simulink model "Final_SEA_Model"  (R2021a)
settings: Solver=VariableStepAuto  StartTime=0.0  StopTime=10  RelTol=1e-3
values from neighbouring files (symbols this model uses):
  B = 0.015    [Project_reading_1.m]
  C = 0.8    [Project_reading_1.m]
  g = 5    [Project_reading_1.m]
  J = 0.0236    [Project_reading_1.m]
  k = 3    [Project_reading_1.m]
  Ks = 18000    [Project_reading_1.m]
  Kt = 1.78    [Project_reading_1.m]
  L = 0.0063    [Project_reading_1.m]
  m = 8    [Project_reading_1.m]
  P = 1    [Project_reading_1.m]
  R = 2.1975    [Project_reading_1.m]
libraries: simulink_extras x2, pid_lib x1
settings Model: Creator=Panda  LastModifiedBy=Panda
settings ConfigComp: PSVerificationMode=BugFinder  PSAutoStubLUT=on

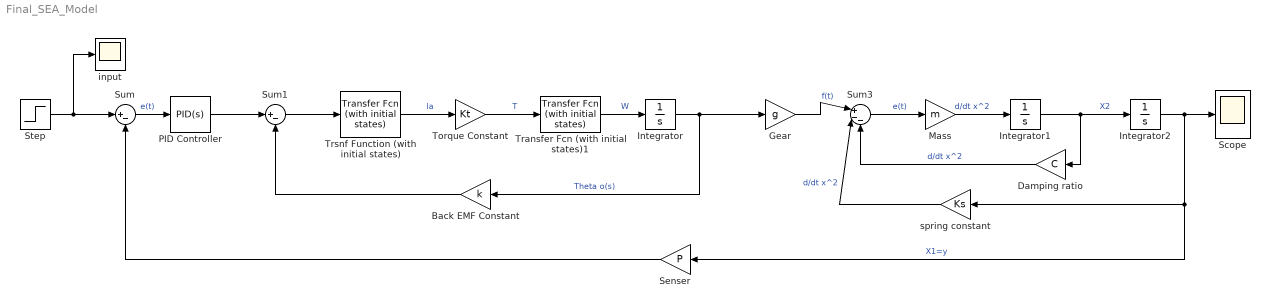
== system Final_SEA_Model ==
  Back EMF Constant : Gain  Gain=k
  Damping ratio : Gain  Gain=C
  Gear : Gain  Gain=g
  Integrator : Integrator
  Integrator1 : Integrator
  Integrator2 : Integrator
  Mass : Gain  Gain=m
  PID Controller : pid_lib/PID Controller  Controller=PID  Form=Parallel  TimeDomain=Continuous-time  UseExternalTs=off  SampleTime=-1  IntegratorMethod=Forward Euler  FilterMethod=Forward Euler  ControllerParametersSource=internal  P=19538.8  I=25686.5  D=2679.99  UseFilter=on  N=100  TunerSelectOption=Transfer Function Based (PID Tuner App)  InitialConditionSource=internal  InitialConditionForIntegrator=0  InitialConditionForFilter=0  DifferentiatorICPrevScaledInput=0  ExternalReset=none  TrackingMode=off  Kt=1  LimitOutput=off  SatLimitsSource=internal  UpperSaturationLimit=inf  LowerSaturationLimit=-inf  LinearizeAsGain=on  AntiWindupMode=none  Kb=1  POutMin=[]  POutMax=[]  IOutMin=[]  IOutMax=[]  DOutMin=[]  DOutMax=[]  NOutMin=[]  NOutMax=[]  SumOutMin=[]  SumOutMax=[]  SaturationOutMin=[]  SaturationOutMax=[]  PParamMin=[]  PParamMax=[]  IParamMin=[]  IParamMax=[]  DParamMin=[]  DParamMax=[]  NParamMin=[]  NParamMax=[]  KbParamMin=[]  KbParamMax=[]  KtParamMin=[]  KtParamMax=[]  KbOutMin=[]  KbOutMax=[]  KtOutMin=[]  KtOutMax=[]  IntegratorOutMin=[]  IntegratorOutMax=[]  FilterOutMin=[]  FilterOutMax=[]  SumI1OutMin=[]  SumI1OutMax=[]  SumI2OutMin=[]  SumI2OutMax=[]  SumI3OutMin=[]  SumI3OutMax=[]  SumI4OutMin=[]  SumI4OutMax=[]  SumDOutMin=[]  SumDOutMax=[]  DifferentiatorOutMin=[]  DifferentiatorOutMax=[]  FilterDiffOutCoefMin=[]  FilterDiffOutCoefMax=[]  ReciprocalOutMin=[]  ReciprocalOutMax=[]  SumDenOutMin=[]  SumDenOutMax=[]  SumNumOutMin=[]  SumNumOutMax=[]  DivideOutMin=[]  DivideOutMax=[]  UdiffTsProdOutMin=[]  UdiffTsProdOutMax=[]  NTsProdOutMin=[]  NTsProdOutMax=[]  UintegralTsProdOutMin=[]  UintegralTsProdOutMax=[]  UngainTsProdOutMin=[]  UngainTsProdOutMax=[]  IntegratorContinuousStateAttributes=''  IntegratorStateMustResolveToSignalObject=off  IntegratorRTWStateStorageClass=Auto  FilterContinuousStateAttributes=''  FilterStateMustResolveToSignalObject=off  FilterRTWStateStorageClass=Auto  ParallelPVariant=InternalParameters  IdealPVariant=Disabled  IVariant=InternalParameters  DVariant=InternalParameters  IntegratorVariant=Continuous  SatVariant=Disabled  AWVariant=Passthrough  PCopyVariant=Disabled  TRVariant=Disabled  FdbkBlocksVariant=Forward  IdealPFdbkVariant=Disabled  SatFdbkVariant=Disabled  DerivativeFilterVariant=ContFilter  NVariant=InternalParameters  NCopyVariant=Disabled  FilterICVariant=InternalICsFilter  IntegratorICVariant=InternalICs  ExternalResetVariant=Disabled  TRSumVariant=Passthrough  SumFdbkVariant=Disabled  SumVariant=Sum_PID  TsampFilterVariant=InternalTs  TsampNgainVariant=Passthrough  TsampIntegralVariant=Passthrough  ExternalSaturationOutDataTypeStr=Inherit: Same as second input
  Scope : Scope
  Senser : Gain  Gain=P
  Step : Step  Time=0  SampleTime=0
  Sum : Sum  Inputs=|+-
  Sum1 : Sum  Inputs=|+-
  Sum3 : Sum  Inputs=|+--
  Torque Constant : Gain  Gain=Kt
  Transfer Fcn (with initial states)1 : simulink_extras/Additional Linear/Transfer Fcn (with initial states)  N=[1]  D="[J  B]"  X0=.5
  Trsnf Function (with initial states) : simulink_extras/Additional Linear/Transfer Fcn (with initial states)  N=[1]  D="[L  R]"  X0=.5
  input : Scope
  spring constant : Gain  Gain=Ks
  wires:
  Trsnf Function (with initial states)/1 -> Torque Constant/1  "la"
  Torque Constant/1 -> Transfer Fcn (with initial states)1/1  "T"
  Sum1/1 -> Trsnf Function (with initial states)/1
  Back EMF Constant/1 -> Sum1/2
  Step/1 -> input/1, Sum/1
  Transfer Fcn (with initial states)1/1 -> Integrator/1  "W"
  Integrator/1 -> Back EMF Constant/1, Gear/1  "Theta o(s)"
  Gear/1 -> Sum3/1  "f(t)"
  Mass/1 -> Integrator1/1  "d/dt x^2"
  Integrator1/1 -> Damping ratio/1, Integrator2/1  "X2"
  Sum3/1 -> Mass/1  "e(t)"
  Integrator2/1 -> Senser/1, spring constant/1, Scope/1  "X1=y"
  Damping ratio/1 -> Sum3/3  "d/dt x^2"
  spring constant/1 -> Sum3/2  "d/dt x^2"
  Senser/1 -> Sum/2
  Sum/1 -> PID Controller/1  "e(t)"
  PID Controller/1 -> Sum1/1
